simulink model "Mesfreq"  (R2019b)
settings: Solver=VariableStepAuto  StartTime=0.0  StopTime=3  MaxStep=0.0001  MinStep=0.0001  RelTol=1e-3
settings Model: Creator=jeanz  LastModifiedBy=jeanz
settings SolverCC: InitialStep=0.0001

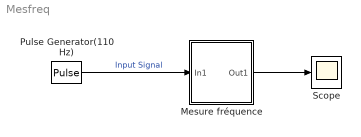
== system Mesfreq ==
  Mesure fréquence : Subsystem
  Pulse Generator(110Hz) : DiscretePulseGenerator  PulseType=Time based  Amplitude=5  Period=1/222  PulseWidth=50
  Scope : Scope
  wires:
  Mesure fréquence/1(Out1) -> Scope/1
  Pulse Generator(110Hz)/1 -> Mesure fréquence/1(In1)  "Input Signal"

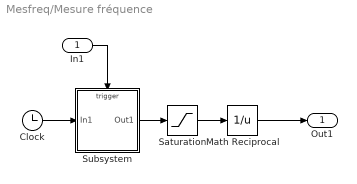
== system Mesfreq/Mesure fréquence ==
  In1 : Inport
  Clock : Clock
  Math Reciprocal : Math  Operator=reciprocal  SaturateOnIntegerOverflow=on
  Saturation : Saturate  UpperLimit=1  LowerLimit=0.003
  Subsystem : Subsystem
  Out1 : Outport
  wires:
  In1/1 -> Subsystem/Trigger
  Clock/1 -> Subsystem/1(In1)
  Subsystem/1(Out1) -> Saturation/1
  Saturation/1 -> Math Reciprocal/1
  Math Reciprocal/1 -> Out1/1

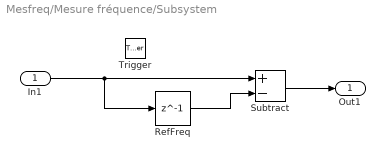
== system Mesfreq/Mesure fréquence/Subsystem ==
  In1 : Inport
  Trigger : TriggerPort  VariantControl=Variant  PortDimensions=1
  RefFreq : Delay  DelayLength=1  InitialCondition=0
  Subtract : Sum  Inputs=+-
  Out1 : Outport
  wires:
  In1/1 -> RefFreq/1, Subtract/1
  RefFreq/1 -> Subtract/2
  Subtract/1 -> Out1/1
